simulink model "Lab3"  (R2022a)
settings: Solver=VariableStepAuto  StartTime=0.0  StopTime=100  RelTol=1e-3
values from neighbouring files (symbols this model uses):
  gamma = 5    [code3.m]
  J = 0.02    [code3.m]
  Kb = 0.015    [code3.m]
  Kf = 2    [code3.m]
  Km = 0.015    [code3.m]
  L = 0.5    [code3.m]
  R = 2    [code3.m]
libraries: slpidlib x1
settings Model: Creator=fades  LastModifiedBy=fades

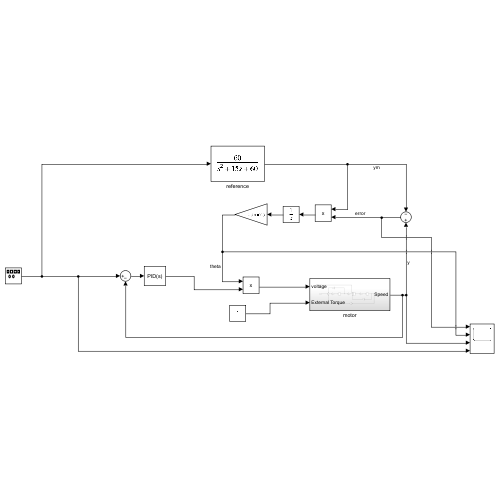
[thumbnail: Simulink's stored preview of the top-level diagram]
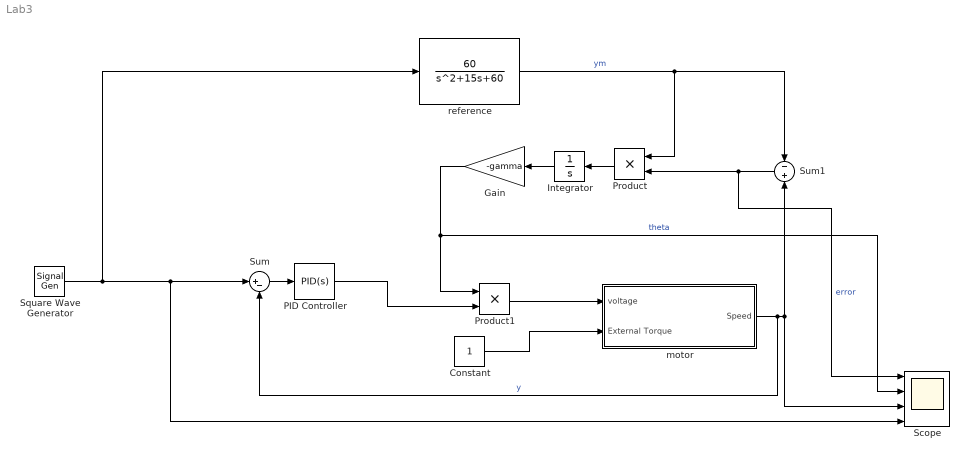
== system Lab3 ==
  Constant : Constant
  Gain : Gain  Gain=-gamma
  Integrator : Integrator
  PID Controller : slpidlib/PID Controller  Controller=PID  Form=Parallel  TimeDomain=Continuous-time  UseExternalTs=off  SampleTime=-1  IntegratorMethod=Forward Euler  FilterMethod=Forward Euler  ControllerParametersSource=internal  P=30  I=100  UseKiTs=off  D=0  N=13.5323447314473  UseFilter=on  TunerSelectOption=Transfer Function Based (PID Tuner App)  InitialConditionSource=internal  InitialConditionForIntegrator=0  InitialConditionForFilter=0  DifferentiatorICPrevScaledInput=0  ExternalReset=none  TrackingMode=off  Kt=1  LimitOutput=off  SatLimitsSource=internal  UpperSaturationLimit=inf  LowerSaturationLimit=-inf  LinearizeAsGain=on  AntiWindupMode=none  Kb=1  POutMin=[]  POutMax=[]  IOutMin=[]  IOutMax=[]  DOutMin=[]  DOutMax=[]  NOutMin=[]  NOutMax=[]  SumOutMin=[]  SumOutMax=[]  SaturationOutMin=[]  SaturationOutMax=[]  PParamMin=[]  PParamMax=[]  IParamMin=[]  IParamMax=[]  DParamMin=[]  DParamMax=[]  NParamMin=[]  NParamMax=[]  KbParamMin=[]  KbParamMax=[]  KtParamMin=[]  KtParamMax=[]  KbOutMin=[]  KbOutMax=[]  KtOutMin=[]  KtOutMax=[]  IntegratorOutMin=[]  IntegratorOutMax=[]  FilterOutMin=[]  FilterOutMax=[]  SumI1OutMin=[]  SumI1OutMax=[]  SumI2OutMin=[]  SumI2OutMax=[]  SumI3OutMin=[]  SumI3OutMax=[]  SumI4OutMin=[]  SumI4OutMax=[]  SumDOutMin=[]  SumDOutMax=[]  DifferentiatorOutMin=[]  DifferentiatorOutMax=[]  FilterDiffOutCoefMin=[]  FilterDiffOutCoefMax=[]  ReciprocalOutMin=[]  ReciprocalOutMax=[]  SumDenOutMin=[]  SumDenOutMax=[]  SumNumOutMin=[]  SumNumOutMax=[]  DivideOutMin=[]  DivideOutMax=[]  UdiffTsProdOutMin=[]  UdiffTsProdOutMax=[]  NTsProdOutMin=[]  NTsProdOutMax=[]  UintegralTsProdOutMin=[]  UintegralTsProdOutMax=[]  UngainTsProdOutMin=[]  UngainTsProdOutMax=[]  IntegratorContinuousStateAttributes=''  IntegratorStateMustResolveToSignalObject=off  IntegratorRTWStateStorageClass=Auto  FilterContinuousStateAttributes=''  FilterStateMustResolveToSignalObject=off  FilterRTWStateStorageClass=Auto  ParallelPVariant=InternalParameters  IdealPVariant=Disabled  IVariant=InternalParameters  DVariant=InternalParameters  IntegratorVariant=Continuous  SatVariant=Disabled  AWVariant=Passthrough  PCopyVariant=Disabled  TRVariant=Disabled  FdbkBlocksVariant=Forward  IdealPFdbkVariant=Disabled  SatFdbkVariant=Disabled  DerivativeFilterVariant=ContFilter  NVariant=InternalParameters  NCopyVariant=Disabled  FilterICVariant=InternalICsFilter  IntegratorICVariant=InternalICs  ExternalResetVariant=Disabled  TRSumVariant=Passthrough  SumFdbkVariant=Disabled  SumVariant=Sum_PID  TsampFilterVariant=InternalTs  TsampNgainVariant=Passthrough  TsampIntegralVariant=Passthrough  ExternalSaturationOutDataTypeStr=Inherit: Same as second input  aMode=0
  Product : Product
  Product1 : Product
  Scope : Scope  NumInputPorts=4
  Square Wave Generator : SignalGenerator  WaveForm=square  Frequency=0.05
  Sum : Sum  Inputs=|+-
  Sum1 : Sum  Inputs=-+
  motor : Subsystem
  reference : TransferFcn  Numerator=[60]  Denominator=[1 15 60]
  wires:
  Constant/1 -> motor/2(External Torque)
  motor/1(Speed) -> Sum/2, Scope/3, Sum1/2  "y"
  Square Wave Generator/1 -> reference/1, Scope/4, Sum/1
  Sum/1 -> PID Controller/1
  reference/1 -> Product/1, Sum1/1  "ym"
  Sum1/1 -> Scope/1, Product/2  "error"
  Product/1 -> Integrator/1
  Integrator/1 -> Gain/1
  Gain/1 -> Scope/2, Product1/1  "theta"
  PID Controller/1 -> Product1/2
  Product1/1 -> motor/1(voltage)

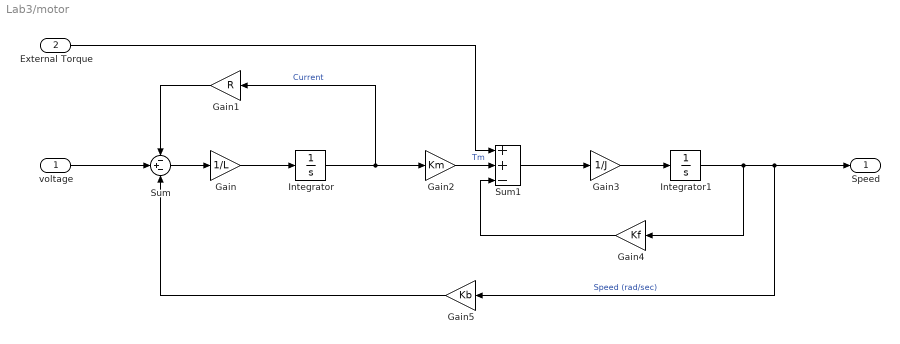
== system Lab3/motor ==
  voltage : Inport
  External Torque : Inport  Port=2
  Gain : Gain  Gain=1/L
  Gain1 : Gain  Gain=R
  Gain2 : Gain  Gain=Km
  Gain3 : Gain  Gain=1/J
  Gain4 : Gain  Gain=Kf
  Gain5 : Gain  Gain=Kb
  Integrator : Integrator
  Integrator1 : Integrator
  Sum : Sum  Inputs=-+-
  Sum1 : Sum  Inputs=++-
  Speed : Outport
  wires:
  Integrator1/1 -> Gain4/1, Speed/1, Gain5/1  "Speed (rad/sec)"
  Gain3/1 -> Integrator1/1
  Sum1/1 -> Gain3/1
  External Torque/1 -> Sum1/1
  voltage/1 -> Sum/2
  Gain2/1 -> Sum1/2  "Tm"
  Integrator/1 -> Gain1/1, Gain2/1  "Current"
  Sum/1 -> Gain/1
  Gain1/1 -> Sum/1
  Gain/1 -> Integrator/1
  Gain4/1 -> Sum1/3
  Gain5/1 -> Sum/3
